simulink model "Model_V5"  (R2024b)
settings: Solver=VariableStepAuto  StartTime=0.0  StopTime=3600*12  RelTol=1e-3
undefined symbols (not defined in the file): PropsSI
libraries: fl_lib x569, SimscapeFluids_lib x61, nesl_utility x27
(part 7 of 7)

== system Model_V5/HVAC/Window (Side) h/Rayleigh Number ==
  g|∆T| : fl_lib/Physical Signals/Functions/PS Gain  gain=9.8066 m/s^2
  gβ|∆T| : fl_lib/Physical Signals/Functions/PS Product
  gβ|∆T| L³ : fl_lib/Physical Signals/Functions/PS Gain  gain=14^3 ft^3
  gβ|∆T| L³/α : fl_lib/Physical Signals/Functions/PS Divide
  gβ|∆T| L³/α/ν : fl_lib/Physical Signals/Functions/PS Divide
  |∆T| : fl_lib/Physical Signals/Nonlinear Operators/PS Abs
      settings: InternalSimscapePortConfiguration="{\"Bottom\":[],\"Left\":[{\"id\":\"I\",\"label\":\"\",\"type\":\"input\"}],\"Right\":[{\"id\":\"O\",\"label\":\"\",\"type\":\"output\"}],\"Top\":[]}"
  ∆T : fl_lib/Physical Signals/Functions/PS Subtract
  β : PMIOPort  Side=Left
  α : PMIOPort  Port=2  Side=Left
  ν : PMIOPort  Port=3  Side=Left
  Ts : PMIOPort  Port=4  Side=Left
  Tair : PMIOPort  Port=5  Side=Left
  Ra : PMIOPort  Port=6  Side=Right
  connections:
  gβ|∆T| L³/α/LConn1 -- gβ|∆T| L³/RConn1
  gβ|∆T|/LConn1 -- β/RConn1
  gβ|∆T| L³/α/ν/LConn1 -- gβ|∆T| L³/α/RConn1
  g|∆T|/LConn1 -- |∆T|/RConn1
  gβ|∆T|/LConn2 -- g|∆T|/RConn1
  |∆T|/LConn1 -- ∆T/RConn1
  gβ|∆T| L³/LConn1 -- gβ|∆T|/RConn1
  gβ|∆T| L³/α/ν/RConn1 -- Ra/RConn1
  gβ|∆T| L³/α/LConn2 -- α/RConn1
  ∆T/LConn2 -- Tair/RConn1
  ∆T/LConn1 -- Ts/RConn1
  ν/RConn1 -- gβ|∆T| L³/α/ν/LConn2
